simulink library "WBToolboxLibrary_repository"  (Simulink 10.0)
settings: Solver=ode45  StartTime=0.0  StopTime=10.0  RelTol=1e-3  EnableMultiTasking=on
undefined symbols (not defined in the file): WBT_modelName, WBT_robotName, WBT_wbiFilename, WBT_wbiList
libraries: simulink x1
(part 2 of 2)

== system WBToolboxLibrary_repository/Model/Jacobians ==
  CentroidalTotalMomentumMatrix : S-Function  FunctionName=BlockFactory  Parameters='CMM', 'WBToolbox', WBTConfigParameters, configBlockAbsName  SFunctionDeploymentMode=off  EnableBusSupport=off  mask(CentroidalTotalMomentumMatrix){}
      mask help:
      | This block retrieves the Centroidal Total Momentum Matrix.
      |
      | Assuming DoFs is the number of internal degrees of freedom of the robot:
      |
      | Input:
      |   - Base pose: 4x4 matrix representing the homogenous transformation between the the base frame and the world frame.
      |   - Joint configuration: Vector of size DoFs, representing the configuration of the joints.
      |
      | Output:
      |   - CMM: a 6x6+dofs matrix representing the Centroidal Momentum Matrix written in the world frame.
      mask init:
      | try
      |     [configBlockAbsName, WBTConfig] = WBToolbox.BlockInitialization(gcb, gcs);
      |     
      |     WBTConfigParameters = WBTConfig.getSimulinkParameters;
      |     clear WBTConfig;
      | catch
      | end
      mask Display:
      | port_label('output', 1, 'CentroidalTotalMomentumMatrix', 'texmode','on')
      | port_label('input', 1, '{}^{world} H_{base}', 'texmode','on')
      | port_label('input', 2, 'Joint configuration')
  DotJNu : Subsystem  mask(DotJNu){frameName='frame'}
      mask prompts: frameName "Frame name"
      mask help:
      | This block computes the product between the time derivative of the Jacobian of the specified frame and the state (base and joints) velocity vector.
      |
      | Assuming DoFs is the number of internal degrees of freedom of the robot:
      |
      | Input:
      |   - Base pose: 4x4 matrix representing the homogenous transformation between the the base frame and the world frame.
      |   - Joint configuration: Vector of size DoFs, representing the configuration of the joints.
      |   - Base velocity: Vector of size 6 representing the linear and angular velocity of the base frame.
      |   - Joints velocity: Vector of size DoFs, representing the velocity of the joints.
      |
      | Output:
      |   - dotJ nu: a 6D vector representing the product between the time derivative of the Jacobian of the specified frame and the state velocity vector
      |
      | Parameters:
      |   - Frame name: the name of the frame. It should be specified in the URDF model.
      mask init: same as WBToolboxLibrary_repository/States/GetMeasurement
      mask DialogControl toggleHighlighting Prompt: Toggle Config Block Highlighting
      mask DialogControl toggleHighlighting Callback:
      | [configBlock, ~] = WBToolbox.BlockInitialization(gcb, gcs);
      | 
      | try
      |     if (strcmp(get_param(configBlock,'HiliteAncestors'),'none'))
      |         hilite_system(configBlock,'find');
      |     else
      |         hilite_system(configBlock,'none');
      |     end
      | catch
      |     error('[%s:ShowConfigBlock:Callback] Failed to process config block name: %s',gcb,configBlock);
      | end
      | 
      | clear configBlock
      mask Display:
      | escapedFrameName = strrep(frameName, '_', '\_');
      | port_label('output', 1, strcat('dot J_{',escapedFrameName,'} \nu'), 'texmode','on')
      | 
      | port_label('input', 1, '{}^{world} H_{base}', 'texmode','on')
      | port_label('input', 2, 'Joint configuration')
      | port_label('input', 3, 'Base velocity')
      | port_label('input', 4, 'Joint velocity')
      | 
      | clear escapedFrameName;
  Jacobian : Subsystem  mask(Jacobian){frameName='frame'}
      mask prompts: frameName "Frame name"
      mask help:
      | This block retrieves the Jacobian of the specified frame.
      |
      | Assuming DoFs is the number of internal degrees of freedom of the robot:
      |
      | Input:
      |   - Base pose: 4x4 matrix representing the homogenous transformation between the the base frame and the world frame.
      |   - Joint configuration: Vector of size DoFs, representing the configuration of the joints.
      |
      | Output:
      |   - Jacobian: a 6x6+dofs matrix representing the Jacobian of the specified frame written in the world frame.
      |
      | Parameters:
      |   - Frame name: the name of the frame. It should be specified in the URDF model.
      mask init: same as WBToolboxLibrary_repository/States/GetMeasurement
      mask DialogControl toggleHighlighting Prompt: Toggle Config Block Highlighting
      mask DialogControl toggleHighlighting Callback:
      | [configBlock, ~] = WBToolbox.BlockInitialization(gcb, gcs);
      | 
      | try
      |     if (strcmp(get_param(configBlock,'HiliteAncestors'),'none'))
      |         hilite_system(configBlock,'find');
      |     else
      |         hilite_system(configBlock,'none');
      |     end
      | catch
      |     error('[%s:ShowConfigBlock:Callback] Failed to process config block name: %s',gcb,configBlock);
      | end
      | 
      | clear configBlock
      mask Display:
      | escapedFrameName = strrep(frameName, '_', '\_');
      | port_label('output', 1, strcat('{}^{world} J_{',escapedFrameName,'}'), 'texmode','on')
      | 
      | port_label('input', 1, '{}^{world} H_{base}', 'texmode','on')
      | port_label('input', 2, 'Joint configuration')
      | 
      | clear escapedFrameName;

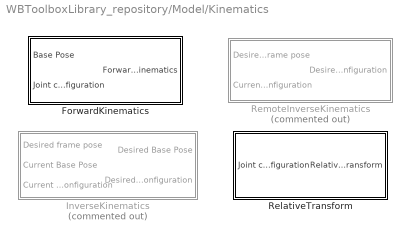
== system WBToolboxLibrary_repository/Model/Kinematics ==
  ForwardKinematics : Subsystem  mask(ForwardKinematics){frameName='frame'}
      mask prompts: frameName "Frame name"
      mask help:
      | This block retrieves the forward kinematics of the specified frame.
      |
      | Assuming DoFs is the number of internal degrees of freedom of the robot:
      |
      | Input:
      |   - Base pose: 4x4 matrix representing the homogenous transformation between the the base frame and the world frame.
      |   - Joint configuration: Vector of size DoFs, representing the configuration of the joints.
      |
      | Output:
      |   - ForwardKinematics: a 4x4 matrix representing the homogenous transformation between the specified frame and the world frame.
      |
      | Parameters:
      |   - Frame name: the name of the frame. It should be specified in the URDF model.
      mask init: same as WBToolboxLibrary_repository/States/GetMeasurement
      mask DialogControl toggleHighlighting Prompt: Toggle Config Block Highlighting
      mask DialogControl toggleHighlighting Callback:
      | [configBlock, ~] = WBToolbox.BlockInitialization(gcb, gcs);
      | 
      | try
      |     if (strcmp(get_param(configBlock,'HiliteAncestors'),'none'))
      |         hilite_system(configBlock,'find');
      |     else
      |         hilite_system(configBlock,'none');
      |     end
      | catch
      |     error('[%s:ShowConfigBlock:Callback] Failed to process config block name: %s',gcb,configBlock);
      | end
      | 
      | clear configBlock
      mask Display:
      | escapedFrameName = strrep(frameName, '_', '\_');
      | % port_label('output', 1, strcat('{}^{world} H_{',escapedFrameName,'}'), 'texmode','on')
      | 
      | port_label('input', 1, '{}^{world} H_{base}', 'texmode','on')
      | port_label('input', 2, 'Joint configuration')
      | 
      | clear escapedFrameName;
  InverseKinematics : Subsystem  Commented=on  InitFcn=|  mask(ForwardKinematics){baseFrame='root_link', endEffFrame='l_sole', optOption=Full Constraint (Position and Orientation), robotName=WBT_robotName, localName=WBT_modelName, wbiFile=WBT_wbiFilename, wbiList=WBT_wbiList}
      | if ~exist('WBT_robotName','var')
      |     WBT_robotName = '';
      | end
      | if ~exist('WBT_modelName','var')
      |     WBT_modelName = 'WBT_simulink';
      | end
      | if ~exist('WBT_wbiFilename','var')
      |     WBT_wbiFilename = 'yarpWholeBodyInterface.ini';
      | end
      | if ~exist('WBT_wbiList','var')
      |     WBT_wbiList = 'ROBOT_TORQUE_CONTROL_JOINTS';
      | end
      mask prompts: baseFrame "Base Frame"; endEffFrame "End Effector frame"; optOption "Optimization Option"; robotName "Robot Port Name"; localName "Model Name"; wbiFile "WBI filename"; wbiList "WBI list name"
      mask help:
      | This block retrieves the forward kinematics of the specified frame.
      |
      | Assuming DoFs is the number of internal degrees of freedom of the robot,
      | Input:
      | - Base pose: 4x4 matrix representing the homogenous transformation between
      |              the the base frame and the world frame.
      | - Joint configuration: Vector of size DoFs, representing the configuration
      |                        of the joints.
      |
      | Output:
      | - ForwardKinematics: a 4x4 matrix representing the homogenous transformation between
      |              the specified frame and the world frame.
      |
      | Parameters:
      | - Frame name: the name of the frame. It should be specified in the URDF model.
      |
      | - Robot Port Name: Name of the ports opened by the robot. (e.g. icub).
      |                    Set an empty string ('') to use the name specified in the
      |                    Whole Body Interface configuration file.
      | - Model Name: Prefix name of the ports opened by the underlying Whole Body Interface.
      | - WBI filename: name of the file containing the configuration of the Whole Body Interface
      | - WBI List Name: name of the list of joints used to configure the Whole Body Interface
      mask TypeOptions optOption: Full Constraint (Position and Orientation) | Position only constraint
      mask Display:
      | escapedBaseFrameName = strrep(baseFrame, '_', '\_');
      | escapedEndEffFrameName = strrep(endEffFrame, '_', '\_');
      | 
      | %port_label('output', 1, strcat('{}^{world} H_{',escapedFrameName,'}'), 'texmode','on')
      | 
      | %port_label('input', 1, '{}^{world} H_{base}', 'texmode','on')
      | %port_label('input', 2, 'Joint configuration')
      | 
      | %clear escapedFrameName;
      | 
      | 
      | % if strcmp(robotPart, 'left')
      | %     prefix = 'l';
      | % else
      | %     prefix = 'r';
      | % end
      | %
      | port_label('input', 1, strcat('{}^{',escapedBaseFrameName,'} H_{',escapedEndEffFrameName,'}^d'), 'texmode','on');
      | 
      | port_label('input', 2, '{}^{world} H_{base}', 'texmode','on')
      | port_label('input', 3, 'q_j', 'texmode','on');
      | %
      | %
      | port_label('output', 1, '{}^{world} H_{base}^d', 'texmode','on')
      | port_label('output', 2, 'q_j^d', 'texmode','on');
  RelativeTransform : Subsystem  mask(RelativeTransform){frame1='frame1', frame2='frame2'}
      mask prompts: frame1 "Frame1 name"; frame2 "Frame2 name"
      mask help:
      | This block calculates the relative transform between two frames.
      |
      | Assuming DoFs is the number of internal degrees of freedom of the robot:
      |
      | Input:
      |   - Joint configuration: Vector of size DoFs, representing the configuration of the joints.
      |
      | Output:
      |   - Transform: a 4x4 matrix representing the homogenous transformation between frame1 and frame2.
      |
      | Parameters:
      |   - Frame1 name: the name of the first frame. It should be part of the URDF model.
      |   - Frame2 name: the name of the second frame. It should be part of the URDF model.
      mask init: same as WBToolboxLibrary_repository/States/GetMeasurement
      mask DialogControl toggleHighlighting Prompt: Toggle Config Block Highlighting
      mask DialogControl toggleHighlighting Callback:
      | [configBlock, ~] = WBToolbox.BlockInitialization(gcb, gcs);
      | 
      | try
      |     if (strcmp(get_param(configBlock,'HiliteAncestors'),'none'))
      |         hilite_system(configBlock,'find');
      |     else
      |         hilite_system(configBlock,'none');
      |     end
      | catch
      |     error('[%s:ShowConfigBlock:Callback] Failed to process config block name: %s',gcb,configBlock);
      | end
      | 
      | clear configBlock
      mask Display:
      | port_label('input', 1, 'Joint configuration')
      | port_label('output', 1, strcat('{}^{', frame1, '}', 'H_{', frame2, '}'), 'texmode','on')
  RemoteInverseKinematics : Subsystem  Commented=on  InitFcn=|  mask(ForwardKinematics){solverName='/cartesianSolver', dofs=12, optOption=Full Constraint (Position and Orientation)}
      | if ~exist('WBT_robotName','var')
      |     WBT_robotName = '';
      | end
      | if ~exist('WBT_modelName','var')
      |     WBT_modelName = 'WBT_simulink';
      | end
      | if ~exist('WBT_wbiFilename','var')
      |     WBT_wbiFilename = 'yarpWholeBodyInterface.ini';
      | end
      | if ~exist('WBT_wbiList','var')
      |     WBT_wbiList = 'ROBOT_TORQUE_CONTROL_JOINTS';
      | end
      mask prompts: solverName "Solver Name"; dofs "#Dofs"; optOption "Optimization Option"
      mask help:
      | This block retrieves the forward kinematics of the specified frame.
      |
      | Assuming DoFs is the number of internal degrees of freedom of the robot,
      | Input:
      | - Base pose: 4x4 matrix representing the homogenous transformation between
      |              the the base frame and the world frame.
      | - Joint configuration: Vector of size DoFs, representing the configuration
      |                        of the joints.
      |
      | Output:
      | - ForwardKinematics: a 4x4 matrix representing the homogenous transformation between
      |              the specified frame and the world frame.
      |
      | Parameters:
      | - Frame name: the name of the frame. It should be specified in the URDF model.
      |
      | - Robot Port Name: Name of the ports opened by the robot. (e.g. icub).
      |                    Set an empty string ('') to use the name specified in the
      |                    Whole Body Interface configuration file.
      | - Model Name: Prefix name of the ports opened by the underlying Whole Body Interface.
      | - WBI filename: name of the file containing the configuration of the Whole Body Interface
      | - WBI List Name: name of the list of joints used to configure the Whole Body Interface
      mask TypeOptions optOption: Full Constraint (Position and Orientation) | Position only constraint
      mask DialogControl Container8 Prompt: Block parameters
      mask Display:
      | disp(solverName)
      | 
      | 
      | 
      | % escapedBaseFrameName = strrep(baseFrame, '_', '\_');
      | % escapedEndEffFrameName = strrep(endEffFrame, '_', '\_');
      | %
      | % %port_label('output', 1, strcat('{}^{world} H_{',escapedFrameName,'}'), 'texmode','on')
      | %
      | % %port_label('input', 1, '{}^{world} H_{base}', 'texmode','on')
      | % %port_label('input', 2, 'Joint configuration')
      | %
      | % %clear escapedFrameName;
      | %
      | %
      | % % if strcmp(robotPart, 'left')
      | % %     prefix = 'l';
      | % % else
      | % %     prefix = 'r';
      | % % end
      | % %
      | 
      | port_label('input', 1, 'H^d', 'texmode','on');
      | % port_label('input', 1, strcat('{}^{',escapedBaseFrameName,'} H_{',escapedEndEffFrameName,'}^d'), 'texmode','on');
      | %
      | % port_label('input', 2, '{}^{world} H_{base}', 'texmode','on')
      | port_label('input', 2, 'q_j(0)', 'texmode','on');
      | % %
      | % %
      | % port_label('output', 1, '{}^{world} H_{base}^d', 'texmode','on')
      | port_label('output', 1, 'q_j^d', 'texmode','on');

== system WBToolboxLibrary_repository/States/GetLimits ==
  S-Function : S-Function  FunctionName=BlockFactory  Parameters='GetLimits','WBToolbox',WBTConfigParameters,configBlockAbsName,limitsType  SFunctionDeploymentMode=off  EnableBusSupport=off
  Min : Outport  VectorParamsAs1DForOutWhenUnconnected=off
  Max : Outport  Port=2  VectorParamsAs1DForOutWhenUnconnected=off
  wires:
  S-Function/1 -> Min/1
  S-Function/2 -> Max/1

== system WBToolboxLibrary_repository/States/GetMeasurement ==
  S-Function : S-Function  FunctionName=BlockFactory  Parameters='GetMeasurement','WBToolbox',WBTConfigParameters,configBlockAbsName,measuredType  SFunctionDeploymentMode=off  EnableBusSupport=off
  Estimate : Outport  VectorParamsAs1DForOutWhenUnconnected=off
  wires:
  S-Function/1 -> Estimate/1

== system WBToolboxLibrary_repository/States/GetMotorMeasurement ==
  S-Function : S-Function  FunctionName=BlockFactory  Parameters='GetMeasurement','WBToolbox',WBTConfigParameters,configBlockAbsName,measuredType  SFunctionDeploymentMode=off  EnableBusSupport=off
  Estimate : Outport  VectorParamsAs1DForOutWhenUnconnected=off
  wires:
  S-Function/1 -> Estimate/1

== system WBToolboxLibrary_repository/Utilities/Configuration ==
  ImConfig : Constant  Value=0
  Terminator : Terminator
  wires:
  ImConfig/1 -> Terminator/1

== system WBToolboxLibrary_repository/Utilities/DampPinv ==
  mat : Inport
  sigma : Inport  Port=2
  Damped Pseudo Inverse : MATLAB Function  TreatAsAtomicUnit=on
  DPinv : Outport  VectorParamsAs1DForOutWhenUnconnected=off
  wires:
  sigma/1 -> Damped Pseudo Inverse/2(sigma)
  Damped Pseudo Inverse/1(DPinv) -> DPinv/1
  mat/1 -> Damped Pseudo Inverse/1(mat)

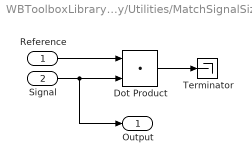
== system WBToolboxLibrary_repository/Utilities/MatchSignalSizes ==
  Reference : Inport
  Signal : Inport  Port=2
  Dot Product : DotProduct  InputSameDT=on  OutDataTypeStr=Inherit: Inherit via internal rule
  Terminator : Terminator
  Output : Outport  VectorParamsAs1DForOutWhenUnconnected=off
  wires:
  Dot Product/1 -> Terminator/1
  Signal/1 -> Output/1, Dot Product/2
  Reference/1 -> Dot Product/1

== system WBToolboxLibrary_repository/Utilities/TruncPinv ==
  S : Inport
  tol : Inport  Port=2
  Truncated PseudoInverse : MATLAB Function  TreatAsAtomicUnit=on
  Tpinv : Outport  VectorParamsAs1DForOutWhenUnconnected=off
  wires:
  S/1 -> Truncated PseudoInverse/1(mat)
  Truncated PseudoInverse/1(TPinv) -> Tpinv/1
  tol/1 -> Truncated PseudoInverse/2(tol)

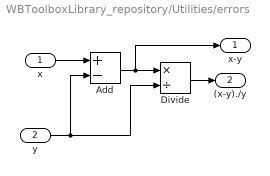
== system WBToolboxLibrary_repository/Utilities/errors ==
  x : Inport
  y : Inport  Port=2
  Add : Sum  Inputs=+-
  Divide : Product  Inputs=*/
  x-y : Outport  VectorParamsAs1DForOutWhenUnconnected=off
  (x-y)./y : Outport  Port=2  VectorParamsAs1DForOutWhenUnconnected=off
  wires:
  Add/1 -> Divide/1, x-y/1
  x/1 -> Add/1
  y/1 -> Add/2, Divide/2
  Divide/1 -> (x-y)./y/1

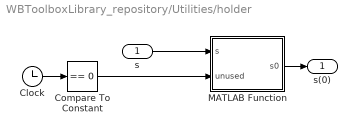
== system WBToolboxLibrary_repository/Utilities/holder  ==
  s : Inport
  Clock : Clock
  Compare To Constant : simulink/Logic and Bit Operations/Compare To Constant  relop===  const=0  OutDataTypeStr=boolean
  MATLAB Function : MATLAB Function  TreatAsAtomicUnit=on
  s(0) : Outport  VectorParamsAs1DForOutWhenUnconnected=off
  wires:
  Clock/1 -> Compare To Constant/1
  MATLAB Function/1(s0) -> s(0)/1
  s/1 -> MATLAB Function/1(s)
  Compare To Constant/1 -> MATLAB Function/2(unused)

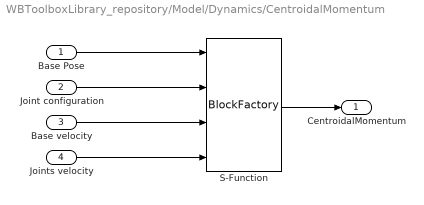
== system WBToolboxLibrary_repository/Model/Dynamics/CentroidalMomentum ==
  Base Pose : Inport
  Joint configuration : Inport  Port=2
  Base velocity : Inport  Port=3
  Joints velocity : Inport  Port=4
  S-Function : S-Function  FunctionName=BlockFactory  Parameters='CentroidalMomentum','WBToolbox',WBTConfigParameters,configBlockAbsName  SFunctionDeploymentMode=off  EnableBusSupport=off
  CentroidalMomentum : Outport  VectorParamsAs1DForOutWhenUnconnected=off
  wires:
  S-Function/1 -> CentroidalMomentum/1
  Base Pose/1 -> S-Function/1
  Joint configuration/1 -> S-Function/2
  Base velocity/1 -> S-Function/3
  Joints velocity/1 -> S-Function/4

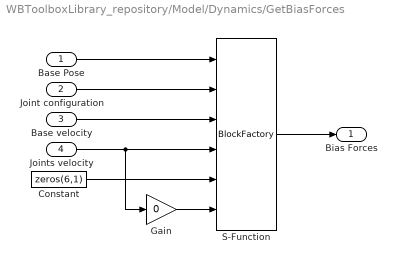
== system WBToolboxLibrary_repository/Model/Dynamics/GetBiasForces ==
  Base Pose : Inport
  Joint configuration : Inport  Port=2
  Base velocity : Inport  Port=3
  Joints velocity : Inport  Port=4
  Constant : Constant  Value=zeros(6,1)
  Gain : Gain  Gain=0
  S-Function : S-Function  FunctionName=BlockFactory  Parameters='InverseDynamics','WBToolbox',WBTConfigParameters,configBlockAbsName  SFunctionDeploymentMode=off  EnableBusSupport=off
  Bias Forces : Outport  VectorParamsAs1DForOutWhenUnconnected=off
  wires:
  S-Function/1 -> Bias Forces/1
  Base Pose/1 -> S-Function/1
  Joint configuration/1 -> S-Function/2
  Base velocity/1 -> S-Function/3
  Joints velocity/1 -> Gain/1, S-Function/4
  Constant/1 -> S-Function/5
  Gain/1 -> S-Function/6

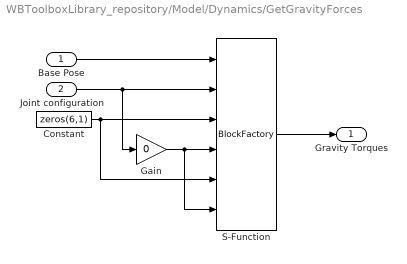
== system WBToolboxLibrary_repository/Model/Dynamics/GetGravityForces ==
  Base Pose : Inport
  Joint configuration : Inport  Port=2
  Constant : Constant  Value=zeros(6,1)
  Gain : Gain  Gain=0
  S-Function : S-Function  FunctionName=BlockFactory  Parameters='InverseDynamics','WBToolbox',WBTConfigParameters,configBlockAbsName  SFunctionDeploymentMode=off  EnableBusSupport=off
  Gravity Torques : Outport  VectorParamsAs1DForOutWhenUnconnected=off
  wires:
  S-Function/1 -> Gravity Torques/1
  Base Pose/1 -> S-Function/1
  Joint configuration/1 -> Gain/1, S-Function/2
  Constant/1 -> S-Function/5, S-Function/3
  Gain/1 -> S-Function/6, S-Function/4

== system WBToolboxLibrary_repository/Model/Dynamics/MassMatrix ==
  Base Pose : Inport
  Joint configuration : Inport  Port=2
  S-Function : S-Function  FunctionName=BlockFactory  Parameters='MassMatrix','WBToolbox',WBTConfigParameters,configBlockAbsName  SFunctionDeploymentMode=off  EnableBusSupport=off
  MassMatrix : Outport  VectorParamsAs1DForOutWhenUnconnected=off
  wires:
  S-Function/1 -> MassMatrix/1
  Base Pose/1 -> S-Function/1
  Joint configuration/1 -> S-Function/2

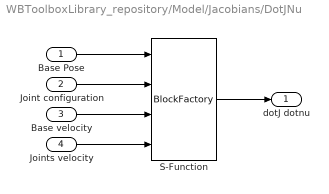
== system WBToolboxLibrary_repository/Model/Jacobians/DotJNu ==
  Base Pose : Inport
  Joint configuration : Inport  Port=2
  Base velocity : Inport  Port=3
  Joints velocity : Inport  Port=4
  S-Function : S-Function  FunctionName=BlockFactory  Parameters='DotJNu','WBToolbox',WBTConfigParameters,configBlockAbsName,frameName  SFunctionDeploymentMode=off  EnableBusSupport=off
  dotJ dotnu : Outport  VectorParamsAs1DForOutWhenUnconnected=off
  wires:
  Joint configuration/1 -> S-Function/2
  Base Pose/1 -> S-Function/1
  S-Function/1 -> dotJ dotnu/1
  Base velocity/1 -> S-Function/3
  Joints velocity/1 -> S-Function/4

== system WBToolboxLibrary_repository/Model/Jacobians/Jacobian ==
  Base Pose : Inport
  Joint configuration : Inport  Port=2
  S-Function : S-Function  FunctionName=BlockFactory  Parameters='Jacobian','WBToolbox',WBTConfigParameters,configBlockAbsName,frameName  SFunctionDeploymentMode=off  EnableBusSupport=off
  ForwardKinematics : Outport  VectorParamsAs1DForOutWhenUnconnected=off
  wires:
  S-Function/1 -> ForwardKinematics/1
  Base Pose/1 -> S-Function/1
  Joint configuration/1 -> S-Function/2

== system WBToolboxLibrary_repository/Model/Kinematics/ForwardKinematics ==
  Base Pose : Inport
  Joint configuration : Inport  Port=2
  S-Function : S-Function  FunctionName=BlockFactory  Parameters='ForwardKinematics','WBToolbox',WBTConfigParameters,configBlockAbsName,frameName  SFunctionDeploymentMode=off  EnableBusSupport=off
  ForwardKinematics : Outport  VectorParamsAs1DForOutWhenUnconnected=off
  wires:
  S-Function/1 -> ForwardKinematics/1
  Base Pose/1 -> S-Function/1
  Joint configuration/1 -> S-Function/2

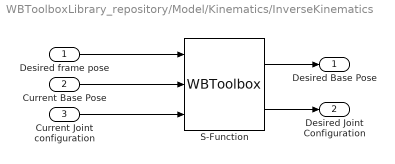
== system WBToolboxLibrary_repository/Model/Kinematics/InverseKinematics ==
  Desired frame pose : Inport
  Current Base Pose : Inport  Port=2
  Current Joint configuration : Inport  Port=3
  S-Function : S-Function  FunctionName=WBToolbox  Parameters='InverseKinematics',robotName,localName,wbiFile,wbiList,baseFrame, endEffFrame,optOption  SFunctionDeploymentMode=off  EnableBusSupport=off
  Desired Base Pose : Outport  VectorParamsAs1DForOutWhenUnconnected=off
  Desired Joint Configuration : Outport  Port=2  VectorParamsAs1DForOutWhenUnconnected=off
  wires:
  S-Function/1 -> Desired Base Pose/1
  Current Base Pose/1 -> S-Function/2
  Current Joint configuration/1 -> S-Function/3
  Desired frame pose/1 -> S-Function/1
  S-Function/2 -> Desired Joint Configuration/1

== system WBToolboxLibrary_repository/Model/Kinematics/RelativeTransform ==
  Joint configuration : Inport
  S-Function : S-Function  FunctionName=BlockFactory  Parameters='RelativeTransform','WBToolbox',WBTConfigParameters,configBlockAbsName,frame1, frame2  SFunctionDeploymentMode=off  EnableBusSupport=off
  RelativeTransform : Outport  VectorParamsAs1DForOutWhenUnconnected=off
  wires:
  S-Function/1 -> RelativeTransform/1
  Joint configuration/1 -> S-Function/1

== system WBToolboxLibrary_repository/Model/Kinematics/RemoteInverseKinematics ==
  Desired frame pose : Inport
  Current Joint configuration : Inport  Port=2
  S-Function : S-Function  FunctionName=WBToolbox  Parameters='RemoteInverseKinematics',solverName, dofs, optOption  SFunctionDeploymentMode=off  EnableBusSupport=off
  Desired Joint Configuration : Outport  VectorParamsAs1DForOutWhenUnconnected=off
  wires:
  S-Function/1 -> Desired Joint Configuration/1
  Desired frame pose/1 -> S-Function/1
  Current Joint configuration/1 -> S-Function/2

== matlab function Utilities/holder /MATLAB Function ==
  data: s input double; s0 output double; unused input double
function s0 = fcn(s, ~)
persistent state
%#codegen

if isempty(state)
    state = s;
end

s0 = state;

== matlab function Utilities/DampPinv/Damped Pseudo Inverse ==
  data: mat input double; DPinv output double; sigma input double
function DPinv  = fcn(mat,sigma)
% Economody size svd of mat
[U,S,V] = svd(mat,'econ');
% Damped version of S with sigma
S(S>sigma)=S(S>sigma)./((S(S>sigma)).^2+sigma^2);
% Damped pseudoinverse
DPinv = V*pinv(S)*U';

== matlab function Utilities/TruncPinv/Truncated PseudoInverse ==
  data: mat input double; TPinv output double; tol input double
function TPinv  = fcn(mat,tol)
%#codegen
[U,S,V] = svd(mat,'econ');
% Setting to zero value
% Setting to 1/S(i,i) singular values greater than tol
 S(S>tol)=1./S(S>tol);
 TPinv = V*pinv(S)*U';
